simulink model "data_collection_HILS"  (R2024a)
settings: Solver=FixedStepAuto  StartTime=0.0  StopTime=inf  FixedStep=0.01  RelTol=1e-3
libraries: robotlib x6, simulink x2, sharedtransform x1, eeGeneralControl x1
settings Model: Creator=hmcl  LastModifiedBy=yjchun
settings OptimizationCC: EnhancedBackFolding=on  PassReuseOutputArgsAs=Individual arguments  ZeroExternalMemoryAtStartup=off  ZeroInternalMemoryAtStartup=off  MaxStackSize=64  OptimizeBlockOrder=speed  DifferentSizesBufferReuse=on  OptimizationCustomize=off  EfficientTunableParamExpr=on
settings DebuggingCC: ParameterTunabilityLossMsg=error
settings HardwareCC: ProdBitPerPointer=32  ProdBitPerSizeT=32  ProdBitPerPtrDiffT=32  ProdLargestAtomicFloat=None  ProdIntDivRoundTo=Undefined  ProdEndianess=Unspecified  ProdWordSize=32  ProdHWDeviceType=Generic->Unspecified (assume 32-bit Generic)
settings RTWCC: Description=Embedded Coder  SystemTargetFile=ert.tlc  HardwareBoard=Robot Operating System (ROS)  TLCOptions="-aInlineSetEventsForThisBaseRateFcn=TLC_FALSE -aSuppressMultiTaskScheduler=TLC_FALSE  -aRateBasedStepFcn=0"  TemplateMakefile=ert_default_tmf  Toolchain=Catkin  TargetLang=C++  GPUComputeCapability=3.5
settings CodeAppCC: ForceParamTrailComments=on  IgnoreCustomStorageClasses=off  OperatorAnnotations=on  SimulinkDataObjDesc=on  SFDataObjDesc=on  InsertBlockDesc=on

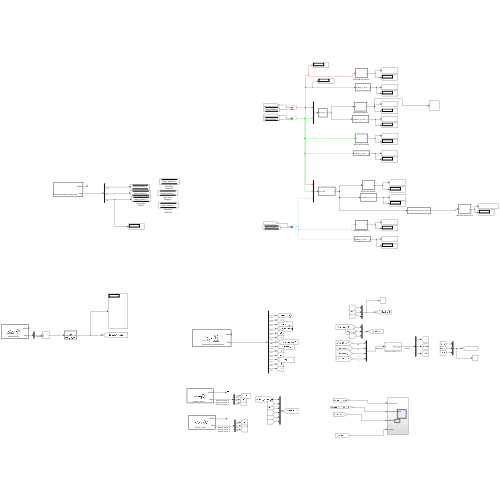
[thumbnail: Simulink's stored preview of the top-level diagram]
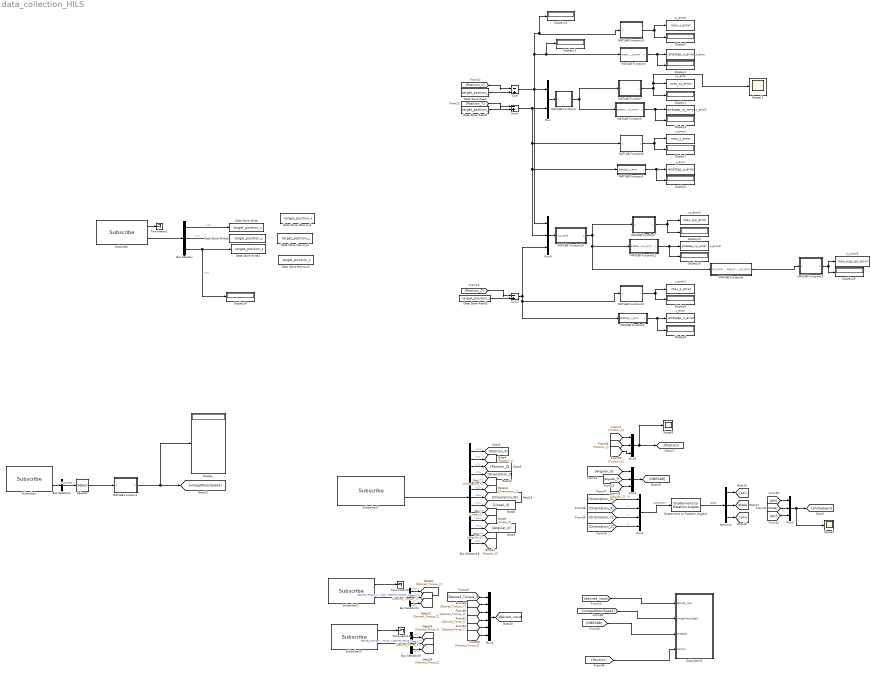
== system data_collection_HILS ==
  Bus Selector : BusSelector  OutputSignals=Pose.Position.X,Pose.Position.Y,Pose.Position.Z
  Bus Selector1 : BusSelector  OutputSignals=Channels
  Bus Selector10 : BusSelector  OutputSignals=X,Y,Z
  Bus Selector11 : BusSelector  OutputSignals=X,Y,Z
  Bus Selector18 : BusSelector  OutputSignals=Pose.Pose.Position.X,Pose.Pose.Position.Y,Pose.Pose.Position.Z,Pose.Pose.Orientation.X,Pose.Pose.Orientation.Y,Pose.Pose.Orientation.Z,Pose.Pose.Orientation.W,Twist.Twist.Linear.X,Twist.Twist.Linear.Y,Twist.Twist.Linear.Z,Twist.Twist.Angular.X,Twist.Twist.Angular.Y,Twist.Twist.Angular.Z
  Data Store Memory3 : DataStoreMemory  DataStoreName=target_position_x  ReadBeforeWriteMsg=warning  WriteAfterWriteMsg=warning  WriteAfterReadMsg=warning  ShowAdditionalParam=off
  Data Store Memory4 : DataStoreMemory  DataStoreName=target_position_y  ReadBeforeWriteMsg=warning  WriteAfterWriteMsg=warning  WriteAfterReadMsg=warning  ShowAdditionalParam=off
  Data Store Memory5 : DataStoreMemory  DataStoreName=target_position_z  ReadBeforeWriteMsg=warning  WriteAfterWriteMsg=warning  WriteAfterReadMsg=warning  ShowAdditionalParam=off
  Data Store Read : DataStoreRead  DataStoreName=target_position_x  IndexOptions=Index vector (dialog)  Indices=1  OutputSizes=1
  Data Store Read1 : DataStoreRead  DataStoreName=target_position_y  IndexOptions=Index vector (dialog)  Indices=1  OutputSizes=1
  Data Store Read3 : DataStoreRead  DataStoreName=target_position_z  IndexOptions=Index vector (dialog)  Indices=1  OutputSizes=1
  Data Store Write : DataStoreWrite  DataStoreName=target_position_x  IndexOptions=Index vector (dialog)  Indices=1  OutputSizes=1
  Data Store Write1 : DataStoreWrite  DataStoreName=target_position_y  IndexOptions=Index vector (dialog)  Indices=1  OutputSizes=1
  Data Store Write2 : DataStoreWrite  DataStoreName=target_position_z  IndexOptions=Index vector (dialog)  Indices=1  OutputSizes=1
  Demux4 : Demux  Outputs=3
  Display{,1..3,5..11,14..16,29} (15 alike) : Display
  MATLAB Function : MATLAB Function  TreatAsAtomicUnit=on
  MATLAB Function1 : MATLAB Function  TreatAsAtomicUnit=on
  MATLAB Function10 : MATLAB Function  TreatAsAtomicUnit=on
  MATLAB Function11 : MATLAB Function  TreatAsAtomicUnit=on
  MATLAB Function12 : MATLAB Function  TreatAsAtomicUnit=on
  MATLAB Function14 : MATLAB Function  TreatAsAtomicUnit=on
  MATLAB Function15 : MATLAB Function  TreatAsAtomicUnit=on
  MATLAB Function2 : MATLAB Function  TreatAsAtomicUnit=on
  MATLAB Function3 : MATLAB Function  TreatAsAtomicUnit=on
  MATLAB Function4 : MATLAB Function  TreatAsAtomicUnit=on
  MATLAB Function5 : MATLAB Function  TreatAsAtomicUnit=on
  MATLAB Function6 : MATLAB Function  TreatAsAtomicUnit=on
  MATLAB Function7 : MATLAB Function  TreatAsAtomicUnit=on
  MATLAB Function8 : MATLAB Function  TreatAsAtomicUnit=on
  MATLAB Function9 : MATLAB Function  TreatAsAtomicUnit=on
  Mux : Mux  Inputs=2
  Mux1 : Mux
  Mux{2..3,5..6} (4 alike) : Mux  Inputs=3
  Mux4 : Mux  Inputs=6
  Quaternions to Rotation Angles1 : sharedtransform/Quaternions to Rotation Angles  rotationOrder=ZYX  aMode=aMode
  Scope11 : Scope
  Scope2 : Scope
  Scope3 : Scope
  Selector : Selector  InputPortWidth=128  IndexOptions=Index vector (dialog)  Indices=1:8  OutputSizes=1
  Subscribe : robotlib/Subscribe  topicSource=Select from ROS network  topic=/mavros/setpoint_position/local  messageType=geometry_msgs/PoseStamped  SampleTime=-1  legacyBusStruct=off  messageQueueLength=1
  Subscribe1 : robotlib/Subscribe  topicSource=Select from ROS network  topic=/mavros/rc/out  messageType=mavros_msgs/RCOut  SampleTime=-1  legacyBusStruct=off  messageQueueLength=1
  Subscribe10 : robotlib/Subscribe  topicSource=Select from ROS network  topic=/thrust_vector  messageType=geometry_msgs/Vector3  SampleTime=-1  legacyBusStruct=off  messageQueueLength=1
  Subscribe11 : robotlib/Subscribe  topicSource=Select from ROS network  topic=/torque_vector  messageType=geometry_msgs/Vector3  SampleTime=-1  legacyBusStruct=off  messageQueueLength=1
  Subscribe17 : robotlib/Subscribe  topicSource=Select from ROS network  topic=/mavros/local_position/odom  messageType=nav_msgs/Odometry  SampleTime=-1  legacyBusStruct=off  messageQueueLength=1
  Subsystem2 : Subsystem
  Sum : Sum  Inputs=|-+
  Sum1 : Sum  Inputs=|-+
  Sum3 : Sum  Inputs=|-+
  Terminator1 : Terminator
  Terminator10 : Terminator
  Terminator11 : Terminator
  x_error : ToWorkspace  VariableName=endstep_x_error  SampleTime=-1
      settings: Save2DSignal=2-D array (concatenate along first dimension)
  x_error1 : ToWorkspace  VariableName=endstep_xy_error  SampleTime=-1
      settings: Save2DSignal=2-D array (concatenate along first dimension)
  x_error2 : ToWorkspace  VariableName=max_y_error  SampleTime=-1
      settings: Save2DSignal=2-D array (concatenate along first dimension)
  x_error3 : ToWorkspace  VariableName=endstep_xyz_error  SampleTime=-1
      settings: Save2DSignal=2-D array (concatenate along first dimension)
  xy_error : ToWorkspace  VariableName=max_xy_error  SampleTime=-1
      settings: Save2DSignal=2-D array (concatenate along first dimension)
  xy_error1 : ToWorkspace  VariableName=max_x_error  SampleTime=-1
      settings: Save2DSignal=2-D array (concatenate along first dimension)
  xy_error2 : ToWorkspace  VariableName=max_xyz_error  SampleTime=-1
      settings: Save2DSignal=2-D array (concatenate along first dimension)
  xy_error3 : ToWorkspace  VariableName=max_avg_xyz_error  SampleTime=-1
      settings: Save2DSignal=2-D array (concatenate along first dimension)
  y_error : ToWorkspace  VariableName=endstep_y_error  SampleTime=-1
      settings: Save2DSignal=2-D array (concatenate along first dimension)
  y_error1 : ToWorkspace  VariableName=max_z_error  SampleTime=-1
      settings: Save2DSignal=2-D array (concatenate along first dimension)
  z_error : ToWorkspace  VariableName=endstep_z_error  SampleTime=-1
      settings: Save2DSignal=2-D array (concatenate along first dimension)
  wires:
  MATLAB Function3/1(y) -> Display6/1, y_error/1
  MATLAB Function2/1(y) -> Display8/1, z_error/1
  MATLAB Function14/1(y) -> xy_error1/1, Display5/1
  MATLAB Function6/1(y) -> x_error2/1, Display7/1
  MATLAB Function/1(y) -> Scope11/1, xy_error/1, Display1/1
  MATLAB Function4/1(y) -> x_error/1, Display2/1
  MATLAB Function11/1(y) -> y_error1/1, Display9/1
  MATLAB Function9/1(y) -> x_error1/1, Display3/1
  Data Store Read/1 -> Sum/2
  Sum3/1 -> MATLAB Function11/1(u), MATLAB Function2/1(endstep_z_error), Mux6/3
  MATLAB Function5/1(y) -> MATLAB Function9/1(endstep_xy_error), MATLAB Function/1(u)
  Data Store Read3/1 -> Sum3/2
  Mux/1 -> MATLAB Function5/1(xy_error)
  Sum/1 -> Mux6/1, MATLAB Function14/1(u), Display10/1, Display11/1, MATLAB Function4/1(endstep_x_error), Mux/1
  Sum1/1 -> Mux6/2, MATLAB Function3/1(endstep_y_error), MATLAB Function6/1(u), Mux/2
  Data Store Read1/1 -> Sum1/2
  [Orientation_W] -> Mux1/1  "W"
  Demux4/3 -> [phi]
  Demux4/1 -> [psi]
  Demux4/2 -> [theta]
  [Orientation_Y] -> Mux1/3  "Y"
  Quaternions to Rotation Angles1/1 -> Demux4/1  "radian"
  [Orientation_X] -> Mux1/2  "x"
  [Orientation_Z] -> Mux1/4  "z"
  Mux1/1 -> Quaternions to Rotation Angles1/1  "quertanion"
  [phi] -> Mux2/1
  Mux2/1 -> Scope2/1, [phithetapsi]
  [psi] -> Mux2/3
  [theta] -> Mux2/2
  [Position_X] -> Sum/1
  [Position_Y] -> Sum1/1
  [Position_Z] -> Sum3/1
  [Angular_X] -> Mux3/1
  [Angular_Y] -> Mux3/2
  [Angular_Z] -> Mux3/3
  Mux3/1 -> [OMEGAB]
  [OMEGAB] -> Subsystem2/3(OMEGAB)
  [desired_input] -> Subsystem2/1(desired_input)
  [omegaMotorSpeed] -> Subsystem2/2(omegaMotorSpeed)
  [Desired_Force_X] -> Mux4/4
  [Desired_Torque_Y] -> Mux4/2
  Bus Selector11/3 -> [Desired_Torque_Z]  "<Z>"
  [Desired_Torque_X] -> Mux4/1
  Subscribe10/1 -> Terminator11/1
  Subscribe11/2 -> Bus Selector11/1  "Desired_Torque_X Desired_Torque_Y Desired_Torque_Z"
  [Desired_Torque_Z] -> Mux4/3
  [Desired_Force_Y] -> Mux4/5
  [Desired_Force_Z] -> Mux4/6
  Subscribe11/1 -> Terminator10/1
  Bus Selector10/3 -> [Desired_Force_Z]  "<Z>"
  Bus Selector10/2 -> [Desired_Force_Y]  "<Y>"
  Subscribe10/2 -> Bus Selector10/1  "Desired_Force_X Desired_Force_Y Desired_Force_Z"
  Bus Selector11/1 -> [Desired_Torque_X]  "<X>"
  Bus Selector11/2 -> [Desired_Torque_Y]  "<Y>"
  Bus Selector10/1 -> [Desired_Force_X]  "<X>"
  Mux4/1 -> [desired_input]
  [Position_X] -> Mux5/1
  [Position_Y] -> Mux5/2
  [Position_Z] -> Mux5/3
  Mux5/1 -> Scope3/1, [Position]
  Mux6/1 -> MATLAB Function10/1(xyz_error)
  MATLAB Function10/1(y) -> MATLAB Function7/1(u), MATLAB Function8/1(xyz_error), MATLAB Function12/1(endstep_xyz_error)
  MATLAB Function7/1(y) -> xy_error2/1, Display15/1
  MATLAB Function12/1(y) -> x_error3/1, Display16/1
  Subscribe17/2 -> Bus Selector18/1
  Bus Selector18/1 -> [Position_X]  "<X>"
  Bus Selector18/2 -> [Position_Y]  "<Y>"
  Bus Selector18/3 -> [Position_Z]  "<Z>"
  Bus Selector18/4 -> [Orientation_X]  "<X>"
  Bus Selector18/5 -> [Orientation_Y]  "<Y>"
  Bus Selector18/6 -> [Orientation_Z]  "<Z>"
  Bus Selector18/7 -> [Orientation_W]  "<W>"
  Bus Selector18/8 -> [Linear_X]  "<X>"
  Bus Selector18/9 -> [Linear_Y]  "<Y>"
  Bus Selector18/10 -> [Linear_Z]  "<Z>"
  Bus Selector18/11 -> [Angular_X]  "<X>"
  Bus Selector18/12 -> [Angular_Y]  "<Y>"
  Bus Selector18/13 -> [Angular_Z]  "<Z>"
  [Position] -> Subsystem2/4(Position)
  MATLAB Function8/1(avg_array_xyz_error) -> MATLAB Function15/1(u)
  MATLAB Function15/1(y) -> xy_error3/1, Display29/1
  Bus Selector/3 -> Display14/1, Data Store Write2/1  "<Z>"
  Bus Selector/1 -> Data Store Write/1  "<X>"
  Subscribe/1 -> Terminator1/1
  Bus Selector/2 -> Data Store Write1/1  "<Y>"
  Subscribe/2 -> Bus Selector/1
  MATLAB Function1/1(rad_s_out) -> Display/1, [omegaMotorSpeed]
  Subscribe1/2 -> Bus Selector1/1
  Selector/1 -> MATLAB Function1/1(pwm_in)
  Bus Selector1/1 -> Selector/1  "<Channels>"

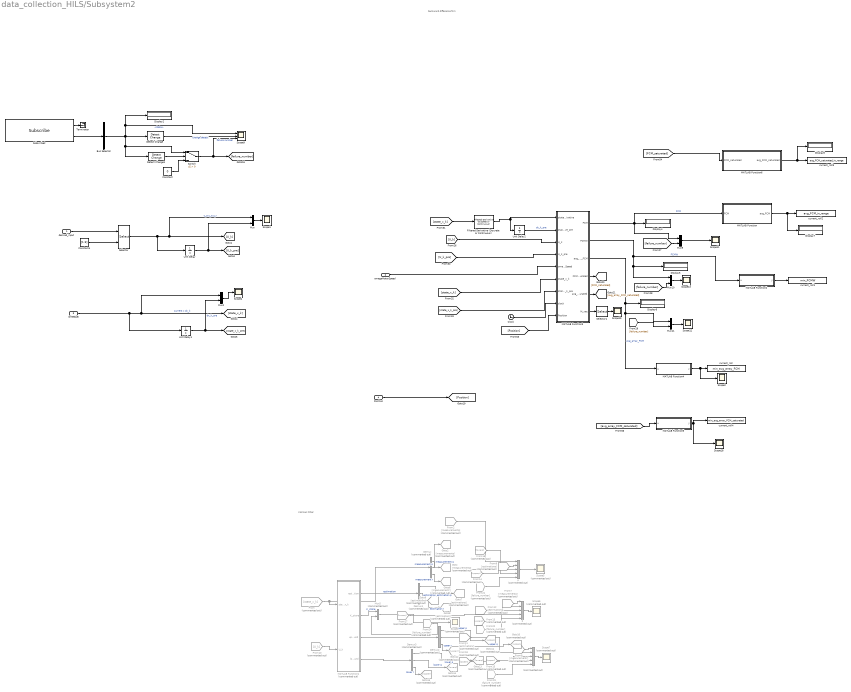
== system data_collection_HILS/Subsystem2 ==
  note: Kalman Filter
  note: backward difference fcm
  desired_input : Inport
  omegaMotorSpeed : Inport  Port=2
  OMEGAB : Inport  Port=3
  Position : Inport  Port=4
  Bus Selector : BusSelector  OutputSignals=Data
  Clock : Clock
  Constant : Constant  Value=0
  Constant4 : Constant  Value=[1:3]
  Demux{,1..3} (4 alike) : Demux  Commented=on  Outputs=3
  Detect Change : simulink/Logic and Bit Operations/Detect Change  vinit=0  OutDataTypeStr=boolean
  Detect Change1 : simulink/Logic and Bit Operations/Detect Change  vinit=0  OutDataTypeStr=boolean
  Display{2,4..8} (6 alike) : Display
  Filtered Derivative (Discrete or Continuous) : eeGeneralControl/Filtered Derivative (Discrete or Continuous)  K=1  T=0.1  B=inf  A=-inf  minRatio=10  init_option=Inherited from block input  x0=0  Ts=-1
      settings: LibrarySourceBlock=|
      | ee_sl_lib/General Control/Filtered Derivative
      | (Discrete or Continuous)
  From : From  Commented=on  GotoTag=state_x_k
  From10 : From  Commented=on  GotoTag=U_k
  From11 : From  Commented=on  GotoTag=estimationr
  From12 : From  Commented=on  GotoTag=estimationq
  From13 : From  Commented=on  GotoTag=upperq
  From14 : From  Commented=on  GotoTag=upperp
  From15 : From  Commented=on  GotoTag=upperr
  From16 : From  Commented=on  GotoTag=lowerp
  From17 : From  Commented=on  GotoTag=lowerq
  From18 : From  Commented=on  GotoTag=lowerr
  From2 : From  Commented=on  GotoTag=measurementp
  From{21..24} (4 alike) : From  Commented=on  GotoTag=failure_number
  From7 : From  Commented=on  GotoTag=measurementq
  From8 : From  Commented=on  GotoTag=measurementr
  From9 : From  Commented=on  GotoTag=estimationp
  Goto : Goto  Commented=on  GotoTag=measurementp
  Goto10 : Goto  Commented=on  GotoTag=upperq
  Goto11 : Goto  Commented=on  GotoTag=upperp
  Goto12 : Goto  Commented=on  GotoTag=upperr
  Goto13 : Goto  Commented=on  GotoTag=lowerp
  Goto14 : Goto  Commented=on  GotoTag=lowerq
  Goto15 : Goto  Commented=on  GotoTag=lowerr
  Goto2 : Goto  Commented=on  GotoTag=measurementq
  Goto6 : Goto  Commented=on  GotoTag=measurementr
  Goto7 : Goto  Commented=on  GotoTag=estimationp
  Goto8 : Goto  Commented=on  GotoTag=estimationr
  Goto9 : Goto  Commented=on  GotoTag=estimationq
  MATLAB Function : MATLAB Function  TreatAsAtomicUnit=on
  MATLAB Function1 : MATLAB Function  Commented=on  TreatAsAtomicUnit=on
  MATLAB Function2 : MATLAB Function  TreatAsAtomicUnit=on
  MATLAB Function3 : MATLAB Function  TreatAsAtomicUnit=on
  MATLAB Function4 : MATLAB Function  TreatAsAtomicUnit=on
  MATLAB Function5 : MATLAB Function  TreatAsAtomicUnit=on
  MATLAB Function6 : MATLAB Function  TreatAsAtomicUnit=on
  Mux{,2,9..11} (5 alike) : Mux  Inputs=2
  Mux5 : Mux  Commented=on  Inputs=2
  Scope{1..2,4,11..13,18..19} (8 alike) : Scope
  Scope{5..8} (4 alike) : Scope  Commented=on
  Scope9 : Scope  NumInputPorts=3
  Selector : Selector  InputPortWidth=6  IndexOptions=Index vector (port)  Indices=[1 3]  OutputSizes=1
  Selector1 : Selector  InputPortWidth=9  IndexOptions=Index vector (dialog)  Indices=[1 5 9]  OutputSizes=1
  Subscribe2 : robotlib/Subscribe  topicSource=Select from ROS network  topic=/mavros/keyboard_command/failure_number  messageType=std_msgs/Float32  SampleTime=-1  legacyBusStruct=off  messageQueueLength=1
  Switch : Switch  Criteria=u2 > Threshold  SaturateOnIntegerOverflow=off  InputSameDT=off
  Terminator : Terminator
  Unit Delay : UnitDelay  SampleTime=-1  HasFrameUpgradeWarning=on
  Unit Delay1 : UnitDelay  SampleTime=-1  HasFrameUpgradeWarning=on
  Unit Delay2 : UnitDelay  SampleTime=-1  HasFrameUpgradeWarning=on
  current_roll : ToWorkspace  VariableName=min_avg_array_FCM  SampleTime=-1
      settings: Save2DSignal=2-D array (concatenate along first dimension)
  current_roll1 : ToWorkspace  VariableName=min_FCMW  SampleTime=-1
      settings: Save2DSignal=2-D array (concatenate along first dimension)
  current_roll2 : ToWorkspace  VariableName=avg_FCM_in_range  SampleTime=-1
      settings: Save2DSignal=2-D array (concatenate along first dimension)
  current_roll3 : ToWorkspace  VariableName=avg_FCM_saturated_in_range  SampleTime=-1
      settings: Save2DSignal=2-D array (concatenate along first dimension)
  current_roll4 : ToWorkspace  VariableName=min_avg_array_FCM_saturated  SampleTime=-1
      settings: Save2DSignal=2-D array (concatenate along first dimension)
  p : Mux  Commented=on  Inputs=5
  q : Mux  Commented=on  Inputs=5
  r : Mux  Commented=on  Inputs=5
  wires:
  desired_input/1 -> Selector/1
  Unit Delay/1 -> Mux/2, [U_k_pre]
  OMEGAB/1 -> Mux2/1, [state_x_k], Unit Delay1/1  "current x dx_k"
  Unit Delay1/1 -> Mux2/2, [state_x_k_pre]  "dx_k_pre"
  Constant4/1 -> Selector/2
  Selector/1 -> Mux/1, [U_k], Unit Delay/1  "u_p u_q u_r"
  Mux/1 -> Scope1/1
  Mux2/1 -> Scope4/1
  Subscribe2/1 -> Terminator/1
  Subscribe2/2 -> Bus Selector/1
  Bus Selector/1 -> Switch/1, Detect Change1/1, Scope9/1, Display2/1, Detect Change/1  "<Data>"
  Detect Change/1 -> Scope9/2  "change detect"
  Detect Change1/1 -> Switch/2
  Switch/1 -> [failure_number], Scope9/3  "failure number"
  Constant/1 -> Switch/3
  [failure_number] -> Mux9/2
  Mux11/1 -> Scope12/1
  MATLAB Function3/2(FCMW) -> Mux10/1, Display5/1, MATLAB Function2/1(u)  "FCMW"
  [state_x_k] -> Filtered Derivative (Discrete or Continuous)/1
  [U_k_pre] -> MATLAB Function3/4(U_k_pre)
  Mux10/1 -> Scope13/1
  [state_x_k] -> MATLAB Function3/6(state_x_k)
  [failure_number] -> Mux10/2
  Mux9/1 -> Scope11/1
  MATLAB Function3/3(avg_array_FCM) -> MATLAB Function4/1(u), Mux11/1, Display6/1  "avg_array_FCM"
  [failure_number] -> Mux11/2
  MATLAB Function3/1(FCM) -> MATLAB Function/1(FCM), Display4/1, Mux9/1  "FCM"
  [U_k] -> MATLAB Function3/3(U_k)
  omegaMotorSpeed/1 -> MATLAB Function3/5(omegaMotorSpeed)
  [state_x_k_pre] -> MATLAB Function3/7(state_x_k_pre)
  Demux1/3 -> Goto8/1  "estimation r"
  MATLAB Function1/1(estimation) -> Demux1/1  "estimation"
  MATLAB Function1/4(lower_bound) -> Demux3/1
  From2/1 -> p/1
  From13/1 -> q/3
  From21/1 -> p/5
  From12/1 -> q/2
  From16/1 -> p/4
  Demux/1 -> Goto/1  "measurement p"
  Demux1/2 -> Goto9/1  "estimation q"
  Demux3/2 -> Goto14/1  "lower q"
  q/1 -> Scope6/1
  From18/1 -> r/4
  Demux1/1 -> Goto7/1  "estimation p"
  r/1 -> Scope7/1
  From23/1 -> r/5
  Demux/2 -> Goto2/1  "measurement q"
  Demux2/2 -> Goto10/1  "upper q"
  From9/1 -> p/2
  From/1 -> Demux/1, MATLAB Function1/1(state_x_k)
  From14/1 -> p/3
  Demux3/3 -> Goto15/1  "lower r"
  Demux3/1 -> Goto13/1  "lower p"
  Demux2/1 -> Goto11/1  "upper p"
  From22/1 -> q/5
  From10/1 -> MATLAB Function1/2(U_k)
  From11/1 -> r/2
  From24/1 -> Mux5/2
  From7/1 -> q/1
  p/1 -> Scope5/1
  From17/1 -> q/4
  MATLAB Function1/3(upper_bound) -> Demux2/1
  Demux/3 -> Goto6/1  "measurement r"
  MATLAB Function1/2(K_store) -> Mux5/1  "K_store"
  From15/1 -> r/3
  Mux5/1 -> Scope8/1
  From8/1 -> r/1
  Demux2/3 -> Goto12/1  "upper r"
  MATLAB Function4/1(y) -> current_roll/1, Scope2/1
  MATLAB Function2/1(y) -> current_roll1/1
  Filtered Derivative (Discrete or Continuous)/1 -> Unit Delay2/1, MATLAB Function3/1(state_derivative)
  MATLAB Function/1(avg_FCM) -> current_roll2/1, Display7/1
  Clock/1 -> MATLAB Function3/8(clock)
  Position/1 -> [Position]
  [FCM_saturated] -> MATLAB Function6/1(FCM_saturated)
  MATLAB Function6/1(avg_FCM_saturated) -> Display8/1, current_roll3/1
  [Position] -> MATLAB Function3/9(Position)
  MATLAB Function3/4(FCM_saturated) -> [FCM_saturated]
  MATLAB Function3/5(avg_array_FCM_saturated) -> [avg_array_FCM_saturated]
  MATLAB Function5/1(y) -> current_roll4/1, Scope18/1
  [avg_array_FCM_saturated] -> MATLAB Function5/1(u)
  MATLAB Function3/6(M_vec) -> Selector1/1
  Selector1/1 -> Scope19/1
  Unit Delay2/1 -> MATLAB Function3/2(state_derivative_pre)  "dx_k_pre"

== matlab function data_collection_HILS/Subsystem2/MATLAB Function ==
  data: FCM input; avg_FCM output
function avg_FCM = fcn(FCM)
% HILS 환경에서는 전체 시뮬레이션 시간 동안의 누적 평균을 계산합니다.

    coder.extrinsic('assignin'); 
    persistent total_sum total_count;

    % persistent 변수 초기화
    if isempty(total_sum)
        total_sum = 0;
    end
    if isempty(total_count)
        total_count = 0;
    end

    % 매 스텝마다 합계와 카운트를 누적
    total_sum = total_sum + FCM;
    total_count = total_count + 1;

    % 현재까지의 평균 계산 (0으로 나누는 오류 방지)
    if total_count > 0
        avg_FCM = total_sum / total_count;
    else
        avg_FCM = 0; % 초기값은 0으로 설정
    end
    
    % 계산된 평균값을 MATLAB Workspace의 'avg_FCM_in_range' 변수에 실시간으로 전송
    assignin('base', 'avg_FCM_in_range', avg_FCM);

end

== matlab function data_collection_HILS/Subsystem2/MATLAB Function1 ==
  data: state_x_k input; estimation output; U_k input; K_store output; upper_bound output; lower_bound output
function [estimation, K_store,upper_bound, lower_bound]  = fcn(state_x_k, U_k)

%% Extended Kalman Filter Example
%% Initial Conditions
coder.extrinsic('delft_evaluate_jacobians');
coder.extrinsic('size');
coder.extrinsic('norm');
coder.extrinsic('eye');
coder.extrinsic('diag');
coder.extrinsic('subs');
coder.extrinsic('calculate_dynamics');
% persistent 변수 선언
persistent initialized xp Pp;

% 초기화가 필요할 때만 실행
if isempty(initialized)
    initialized = true; % 초기화 완료 표시
    xp = state_x_k;    % guess of initial posteriori estimation
    Pp = 100*eye(3); % guess of initial error covariance
    sigma_Pp = sqrt(diag(Pp));
    three_sigma = zeros(3,1);
    upper_bound = zeros(3,1);
    lower_bound = zeros(3,1);

    P = zeros(3,3);


    x_ = zeros(3,1);
    P_ = zeros(3,3);
    Pp_ = zeros(3,3);
    F = zeros(3,3);
    Q = zeros(3,3);
    R = zeros(3,3);
    K = zeros(3,3);
    H = zeros(3,3);
    I = zeros(3,3);
    estimation = zeros(3,1);
    K_store = zeros(1,1);
    disp('initialized.');
end

p = xp(1);
q = xp(2);
r = xp(3);

u_p = U_k(1);
u_q = U_k(2);
u_r = U_k(3);

sigma_w = 0.1;      % system noise (std of acceleration)
sigma_v = 0.2;      % measurement noise (std of position sensor)
Q = diag([sigma_w^2 sigma_w^2 sigma_w^2]); % system noise covariance matrix
R = diag([sigma_v^2 sigma_v^2 sigma_v^2]); % measurement noise covariance matrix
%% Dynamics
% system matrix

Gamma = [1 0 0;0 1 0;0 0 1];      % Gamma (related to system noise)
H = [1 0 0;0 1 0;0 0 1];          % Measurement matrix

%% KF Routine
    %% True dynamics
    % x(:,i+1) = [sin(x(2,i)*(i)) + randn*sigma_w; x(2,i) ]; % system dynamics
    % x = double(subs(F, {'p', 'q', 'r','u_p', 'u_q', 'u_r'},{p, q, r, u_p, u_q, u_r}));
    %% ====================================================
    %% Time update
    %% ====================================================
    %% Equation 1: Prediction of state
    % x_ = [sin(xp(2,i)*(i)); xp(2,i)];
    x_ = calculate_dynamics(p, q, r, u_p, u_q, u_r);
    %% compute Jacobian
    % F = [0 (i)*cos(x_(2)*(i));
    %     0 1];
    [F_, G_] = delft_evaluate_jacobians(p, q, r, u_p, u_q, u_r);
    %% Equation 2: Prediction of covariance
    F = F_;
    Pp_ = Pp;
    P_ = F*Pp_*F' + Gamma*Q*Gamma';
    %% ====================================================
    %% Measurement update
    %% ====================================================
    %% measurement generation
    % y(i) = H*x(:,i+1) + randn*sigma_v;
    y = state_x_k;
    %% Equation 3: Innovation Covariance
    S = H*P_*H'+R;
    %% Equation 4:  Residual
    nu = y-H*x_;
    %% Equation 5: Kalman gain
    K = P_*H'*S^-1;
    %% Equation 6: State update
    xp = x_ + K * nu;
    estimation = xp;
    %% Equation 7: Covariance update
    I = eye(size(K*H));
    Pp = (I-K*H)*P_;
    %% =====================================================
    %% storing error covariance for ploting
    sigma_Pp = sqrt(diag(Pp));
    % disp('sigma_Pp');
    % disp(size(sigma_Pp));
    three_sigma = 3 * sigma_Pp;
    upper_bound = xp + three_sigma;
    lower_bound = xp - three_sigma;
    %% storing Kalman gain for ploting
    K_store = norm(K);


    
%     %% Plot: position estimate x_1
% figure(1); clf; hold on;
% plot(t,x(1,:),'-b');                  % plot the real plant behavior
% plot(t(1:end-1),y,'.m');                       % plot the observations over this plant
% plot(t,xp(1,:),'-r');                 % plot the Kalman filter prediction over the plant
% plot(t,xp(1,:)+3*sigma_Pp(1,:),':k');  % The threshold in which the true state is
% plot(t,xp(1,:)-3*sigma_Pp(1,:),':k');
% xlabel('time, s'); ylabel('x1: m')
% legend('real','observation','KF','threshold')
% axis([-inf inf -10 10])
% %% Plot: velocity estimate x_2
% figure(2); clf; hold on;
% plot(t,x(2,:),'-b');                  % plot the real plant behavior
% plot(t,xp(2,:),'-r');                 % plot the Kalman filter prediction over the plant
% plot(t,xp(2,:)+3*sigma_Pp(2,:),':k');   % These two are the threshold in witch I'm certain that the plant state is at a given time
% plot(t,xp(2,:)-3*sigma_Pp(2,:),':k');
% xlabel('time, s'); ylabel('x2: rad/s')
% legend('true','KF','threshold')
% axis([-inf inf -5 20])
% %% Plot: Kalman gain norm
% figure(3);
% plot(t(1:end-1),K_store);
% xlabel('time, s'); ylabel('Kalman gain norm')

end

== matlab function data_collection_HILS/Subsystem2/MATLAB Function2 ==
  data: u input; y output
function y = fcn(u)
    coder.extrinsic('assignin');
    persistent min_val; % 최솟값을 저장할 변수

    if isempty(min_val)
        min_val = inf; % 처음에 매우 큰 값으로 초기화
    end

    % 현재 u의 절대값이 기록된 최솟값보다 작으면 업데이트
    if abs(u) < min_val
        min_val = abs(u);
    end

    y = min_val; % 현재까지의 최솟값을 출력
    assignin('base', 'min_avg_array_FCM_saturated', y);
end

== matlab function data_collection_HILS/Subsystem2/MATLAB Function3 ==
  settings: updateMethod=DISCRETE
  data: state_derivative input; state_derivative_pre input; U_k input; U_k_pre input; FCM output; omegaMotorSpeed input; state_x_k input; state_x_k_pre input; FCMW output; avg_array_FCM output; clock input; Position input; FCM_saturated output; avg_array_FCM_saturated output; window_size_ parameter; M_vec output size=9
function [FCM, FCMW, avg_array_FCM, FCM_saturated, avg_array_FCM_saturated,M_vec]  = fcn(state_derivative,state_derivative_pre,U_k,U_k_pre,omegaMotorSpeed,state_x_k,state_x_k_pre,clock, Position, window_size_)
%#codegen

% X_k = current
% X_k_pre = previous
disp('clock = ');
disp(clock);

coder.extrinsic('size');
coder.extrinsic('ctrb');
coder.extrinsic('rank');
coder.extrinsic('inv');
coder.extrinsic('sign');
coder.extrinsic('evalin');
coder.extrinsic('diff');
coder.extrinsic('addpath');
% addpath('/home/hmcl/PX4_testbed/gp_matlab/octo_model');

coder.extrinsic('delft_evaluate_jacobians.m');
coder.extrinsic('calculate_FCMW.m');
coder.extrinsic('calculate_FCMW_saturated.m')

% persistent 변수 선언
persistent initialized avg_array_FCM_ avg_array_FCM_saturated_;
persistent M_prev;

if isempty(M_prev)
    M_prev = eye(3);
end


dt = 0.004; % 시간 간격 % 가제보는 dt = 0.004 로 데이터를 전송및 한다
omega_max = 425.47; % 최대 회전 속도 rad/s, maxRotVelocity in sdf
tau = 0.01; % 액추에이터 시간 상수
M = eye(3);
% window_size_ = 100;

delft_df_dx = zeros(length(state_x_k), length(state_x_k));
delft_df_du = zeros(length(state_x_k), length(U_k));
del_umax = zeros(3,1);
del_uc = zeros(3,1);
signMask = zeros(1,8);
refOmega = zeros(8,1);
signError = zeros(1,1);
rank_con = 0;


rotorMapping = [-1 -1 1;
    1 1 1;
    -1 -1 -1;
    -1 1 -1;
    1 -1 -1;
    1 1 -1;
    1 -1 1;
    -1 1 1];

% rotorMapping = rotorMapping *-1; 

% x = state_x_k1(1);
% y = state_x_k1(2);
% z = state_x_k1(3);
% u = state_x_k1(4);
% v = state_x_k1(5);
% w = state_x_k1(6);
% phi = state_x_k1(7);
% theta = state_x_k1(8);
% psi = state_x_k1(9);
p = state_x_k(1);
q = state_x_k(2);
r = state_x_k(3);

u_p = U_k(1);
u_q = U_k(2);
u_r = U_k(3);

x = Position(1);
y = Position(2);
z = Position(3);



% 초기화가 필요할 때만 실행
if isempty(initialized)
    initialized = true; % 초기화 완료 표시
    FCMW = 1;
    avg_array_FCM = 1.0;
    avg_array_FCM_ = 1.0;

    FCMW_saturated = 1;
    avg_array_FCM_saturated = 1.0;
    avg_array_FCM_saturated_ = 1.0;
    disp('initialized.');
end

disp('-----------------');
% 심볼릭 야코비안 행렬 평가
[df_dx_temp, df_du_temp] = delft_evaluate_jacobians(p, q, r, u_p, u_q, u_r);

% 외부 함수로부터 받은 값을 MATLAB 배열로 변환
delft_df_dx = df_dx_temp; %delft_df_dx = A %3by3   %length(X_k1) by length(X_k1)

delft_df_du = df_du_temp; %delft_df_du = B %3by3    %length(X_k1) by length(U_k1)

A = delft_df_dx;
B = delft_df_du;

debug_info = struct(); 
debug_info.clock = clock;
debug_info.A = A;
debug_info.B_initial = B; 

% 상태 및 입력 차이 계산
diffrate = state_x_k - state_x_k_pre;  % dx는 3x1
du = U_k - U_k_pre;  % du는 3x1

diff_ratedot = state_derivative - state_derivative_pre;




% disp('A = ')
% disp(A)
% disp('du = ')
% disp(du)

% dx_dot = df_dx * dx + df_du * du;
%{
state X 가 정확값이라고 했을때 state X를 미분하면 dx_dot 이 나오게 된다.
그리고 식(6)을 보면 dx_dot 을 근사한 식인 A * dx + B * du 가 있다.
만약 근사한식이 너무 정확하면 dx_dot - (A * dx + B * du) 을 했을때 0 이 된다.
즉, 근사한 식이 정확하면 미분한 식(dx_dot) - 근사한식(A * dx + B * du) 이 0이 되야한다.

하지만 근사한식이 당연히 정확할수 없기 때문에 error가 생기는데
이 에러를 보상해주기 위해, 또는 0으로 수렴 시키기 위해서
del_uc를 정의 해준다.
del_uc는 inv(B) *error 이다.

그래서 dx_dot - (A * dx + B * du + del_uc) 식(11)이 나오고 이 식은 0으로 점점 수렴하게 된다.
%}

error = diff_ratedot - A * diffrate;
debug_info.ER = error; % M 계산에 사용되는 error

M = M_prev; 

% corrcoef_result = corrcoef(state_derivative, A * dx + B * du);
corrcoef_result = corrcoef(diff_ratedot, B * du);

disp('error = ')
disp(error);
disp('B * du = ')
disp(B * du);

for i = 1:3
    if ~isnan(corrcoef_result(1,2))
        M(i, i) = max(corrcoef_result(1,2), 0.001); % 최소값 설정
    else
        M(i, i) = 1;
    end
end
debug_info.corrcoef_result = corrcoef_result;                                                 
debug_info.M = M;

% disp('ER = ')
% disp(error)
% disp('M = ');
% disp(M);
M_vec = M(:);

disp('corrcoef_result = ')
disp(corrcoef_result);

% disp('B = ')
% disp(B)

B = B * M;
debug_info.B_updated = B; % M을 곱한 후 B


M_prev = M;

% disp('B = ')
% disp(B)


% disp('A * dx + B * du = ');
% disp(A * diffrate + B * du);

err = error - B * du; %error : 3by1
% disp('error = ');
% disp(err);
debug_info.err_final = err; % del_uc 계산에 사용되는 최종 error

if (abs(err) == 0)
    
    disp('error is zero');
    FCM = 1;
    FCMW = 1;
    FCM_saturated = 1;

    FCMW_saturated = 1;
    avg_array_FCM = avg_array_FCM_;
    avg_array_FCM_saturated = avg_array_FCM_saturated_;
    return

else
    del_uc = (inv(B)) * err; % del_uc는 3x1
debug_info.del_uc_abs = abs(del_uc);


    rotorMapping_T = rotorMapping'; % 이건 필수인듯?



    % error의 부호를 계산
    for i = 1:length(err)

        signError = sign(err(i));

        signMask = signError .* rotorMapping_T(i,:); % sign(error)를 대체
 

        for j = 1:length(signMask)
            if signMask(j) < 0
                refOmega(j) = omega_max; % signMask가 0보다 작으면 omega_max 할당
            else
                refOmega(j) = 0;         % signMask가 0 이상이면 0 할당
            end
        end

   

        % omegaMotorSpeed [rad/s]
        maxDiff = abs(abs(double(omegaMotorSpeed)) - refOmega); %maxDiff  8by1
  

        % Δu_MAX
        del_umax(i,1) = dt * (1/tau) * sum(maxDiff);

    end
        debug_info.del_umax = del_umax;



    controllability_matrix = ctrb(A,B);
    % disp('controllability_matrix = ')
    % disp(controllability_matrix)

    % 랭크 계산
    rank_con = rank(controllability_matrix);
debug_info.rank = rank_con;

    n = length(A);

 

    if rank_con < n || any(del_umax < abs(del_uc))
        FCM = 0;
    else
        FCM = 1;
    end

if FCM == 0
    fprintf('\n--- FCM=0 DETECTED (Clock: %f) ---\n', debug_info.clock);
    disp('Initial A Matrix:');
    disp(debug_info.A);
    disp('Initial B Matrix:');
    disp(debug_info.B_initial);
    disp('ER (for M calculation):');
    disp(debug_info.ER)

      disp('corrcoef_result:');
    disp(debug_info.corrcoef_result)
    
    disp('Calculated M Matrix:');
    disp(debug_info.M);
    disp('Updated B Matrix (B*M):');
    disp(debug_info.B_updated);
    disp('Final Error (for del_uc):');
    disp(debug_info.err_final);
    disp('Required Control |del_uc|:');
    disp(debug_info.del_uc_abs);
    disp('Max Available Control |del_umax|:');
    disp(debug_info.del_umax);
    disp('Controllability Matrix Rank:');
    disp(debug_info.rank);
    fprintf('-------------------------------------\n\n');
end



    [FCMW_, avg_array_FCM_] = calculate_FCMW(FCM,window_size_);

    FCMW = FCMW_;
    avg_array_FCM = avg_array_FCM_;



    if sqrt(x^2 + y^2) < 10
        FCM_saturated = FCM;
    else
        FCM_saturated = 0;
    end

    [FCMW_saturated_, avg_array_FCM_saturated_] = calculate_FCMW_saturated(FCM_saturated,window_size_);

    FCMW_saturated = FCMW_saturated_;
    avg_array_FCM_saturated = avg_array_FCM_saturated_;


end % if end

disp('-----------------');

end

== matlab function data_collection_HILS/MATLAB Function10 ==
  data: xyz_error input; y output
function y = two_norm(xyz_error)
    coder.extrinsic('norm'); % MATLAB 함수 사용을 알림
    
    

    
    % 'y'를 명확히 초기화
    y = 0; 
    
y = norm(xyz_error,2);

== matlab function data_collection_HILS/MATLAB Function11 ==
  data: u input; y output
function y = fcn(u)
% HILS 환경에서는 전체 시뮬레이션 시간 동안 u의 최댓값을 찾습니다.

    coder.extrinsic('assignin');
    persistent max_val; % 최댓값을 저장할 변수

    % persistent 변수 초기화
    if isempty(max_val)
        max_val = -inf; % 처음에 매우 작은 값으로 초기화
    end

    % 현재 u가 기록된 최댓값보다 크면 업데이트
    if u > max_val
        max_val = u;
    end

    y = max_val; % 현재까지의 최댓값을 출력
    
    % 계산된 최댓값을 MATLAB Workspace 변수에 실시간으로 전송
    assignin('base', 'max_z_error', y);

end

== matlab function data_collection_HILS/MATLAB Function12 ==
  data: endstep_xyz_error input; y output
function y = fcn(endstep_xyz_error)

% z_error 값을 기본 워크스페이스에 저장
assignin('base', 'endstep_xyz_error', endstep_xyz_error);

% 저장된 값을 반환
y = endstep_xyz_error;

end

== matlab function data_collection_HILS/MATLAB Function14 ==
  data: u input; y output
function y = fcn(u)
% HILS 환경에서는 전체 시뮬레이션 시간 동안 u의 최댓값을 찾습니다.

    coder.extrinsic('assignin');
    persistent max_val; % 최댓값을 저장할 변수

    % persistent 변수 초기화
    if isempty(max_val)
        max_val = -inf; % 처음에 매우 작은 값으로 초기화
    end

    % 현재 u가 기록된 최댓값보다 크면 업데이트
    if u > max_val
        max_val = u;
    end

    y = max_val; % 현재까지의 최댓값을 출력
    
    % 계산된 최댓값을 MATLAB Workspace 변수에 실시간으로 전송
    assignin('base', 'max_x_error', y);

end

== matlab function data_collection_HILS/Subsystem2/MATLAB Function5 ==
  data: u input; y output
function y = fcn(u)
% HILS 환경에서는 전체 시뮬레이션 시간 동안 u의 절대값 최솟값을 찾습니다.

    coder.extrinsic('assignin');
    persistent min_val; % 최솟값을 저장할 변수

    % persistent 변수 초기화
    if isempty(min_val)
        min_val = inf; % 처음에 매우 큰 값으로 초기화
    end

    % 현재 u의 절대값이 기록된 최솟값보다 작으면 업데이트
    if abs(u) < min_val
        min_val = abs(u);
    end

    y = min_val; % 현재까지의 최솟값을 출력
    
    % 계산된 최솟값을 MATLAB Workspace 변수에 실시간으로 전송
    assignin('base', 'min_avg_array_FCM_saturated', y);

end

== matlab function data_collection_HILS/Subsystem2/MATLAB Function6 ==
  data: FCM_saturated input; avg_FCM_saturated output
function avg_FCM_saturated = fcn(FCM_saturated)
% HILS 환경에서는 전체 시뮬레이션 시간 동안의 누적 평균을 계산합니다.

    coder.extrinsic('assignin'); 
    persistent total_sum total_count;

    % persistent 변수 초기화
    if isempty(total_sum)
        total_sum = 0;
    end
    if isempty(total_count)
        total_count = 0;
    end

    % 매 스텝마다 합계와 카운트를 누적
    total_sum = total_sum + FCM_saturated;
    total_count = total_count + 1;

    % 현재까지의 평균 계산 (0으로 나누는 오류 방지)
    if total_count > 0
        avg_FCM_saturated = total_sum / total_count;
    else
        avg_FCM_saturated = 0; % 초기값은 0으로 설정
    end
    
    % 계산된 평균값을 MATLAB Workspace 변수에 실시간으로 전송
    assignin('base', 'avg_FCM_saturated_in_range', avg_FCM_saturated);

end

== matlab function data_collection_HILS/MATLAB Function8 ==
  settings: updateMethod=DISCRETE
  data: xyz_error input; window_size_ parameter; avg_array_xyz_error output
function avg_array_xyz_error  = fcn(xyz_error, window_size_)

coder.extrinsic('calculate_xyzerror.m');

% persistent 변수 선언
persistent initialized avg_array_xyz_error_;

% 초기화가 필요할 때만 실행
if isempty(initialized)
    initialized = true; % 초기화 완료 표시
    one_or_zero = 0;
    one_or_zero_ = 0;
    avg_array_xyz_error = 0.0;
    avg_array_xyz_error_ = 0.0;

    disp('initialized.');
end


[one_or_zero_, avg_array_xyz_error_] = calculate_xyzerror(xyz_error,window_size_);

one_or_zero = one_or_zero_;
avg_array_xyz_error = avg_array_xyz_error_;





end

== matlab function data_collection_HILS/MATLAB Function15 ==
  data: u input; y output
function y = fcn(u)
% HILS 환경에서는 전체 시뮬레이션 시간 동안 u의 최댓값을 찾습니다.

    coder.extrinsic('assignin');
    persistent max_val; % 최댓값을 저장할 변수

    % persistent 변수 초기화
    if isempty(max_val)
        max_val = -inf; % 처음에 매우 작은 값으로 초기화
    end

    % 현재 u가 기록된 최댓값보다 크면 업데이트
    if u > max_val
        max_val = u;
    end

    y = max_val; % 현재까지의 최댓값을 출력
    
    % 계산된 최댓값을 MATLAB Workspace 변수에 실시간으로 전송
    assignin('base', 'max_avg_xyz_error', y);

end

== matlab function data_collection_HILS/MATLAB Function1 ==
  data: pwm_in input; rad_s_out output
function rad_s_out = pwm_to_rads(pwm_in)
%#codegen

% 이 함수는 8x1 배열의 PWM 값을 입력받아
% 각 값을 rad/s 단위의 각속도로 변환합니다.

% --- 사용자 정의 파라미터 ---
% Gazebo SDF 파일 또는 PX4 파라미터에 맞춰 수정하세요.
maxRotVelocity = 425.47;  % rad/s
PWM_MIN = 1100;           % 시동(Armed) 시 최소 PWM 값
PWM_MAX = 2200;           % 최대 PWM 값
% -------------------------

% 출력 변수를 8x1 크기의 double 타입 배열로 초기화합니다.
rad_s_out = zeros(8, 1);

% 8개의 채널에 대해 반복 계산합니다.
for i = 1:8
    % 현재 채널의 PWM 값을 가져옵니다.
    % Simulink 입력은 종종 double 타입이므로, 먼저 double로 변환해줍니다.
    pwm_value = double(pwm_in(i));
    
    % 1. PWM 값을 0.0 ~ 1.0 사이의 정규화된 입력으로 변환
    % (pwm_value - PWM_MIN)이 음수가 되지 않도록 saturate 처리
    if pwm_value < PWM_MIN
        normalized_input = 0.0;
    elseif pwm_value > PWM_MAX
        normalized_input = 1.0;
    else
        normalized_input = (pwm_value - PWM_MIN) / (PWM_MAX - PWM_MIN);
    end
    
    % 2. 정규화된 입력을 rad/s로 변환
    rad_s_out(i) = normalized_input * maxRotVelocity;
end

end

== matlab function data_collection_HILS/MATLAB Function ==
  data: u input; y output
function y = fcn(u)
% HILS 환경에서는 전체 시뮬레이션 시간 동안 u의 최댓값을 찾습니다.

    coder.extrinsic('assignin');
    persistent max_val; % 최댓값을 저장할 변수

    % persistent 변수 초기화
    if isempty(max_val)
        max_val = -inf; % 처음에 매우 작은 값으로 초기화
    end

    % 현재 u가 기록된 최댓값보다 크면 업데이트
    if u > max_val
        max_val = u;
    end

    y = max_val; % 현재까지의 최댓값을 출력
    
    % 계산된 최댓값을 MATLAB Workspace 변수에 실시간으로 전송
    assignin('base', 'max_xy_error', y);

end

== matlab function data_collection_HILS/MATLAB Function2 ==
  data: endstep_z_error input; y output
function y = fcn(endstep_z_error)

% z_error 값을 기본 워크스페이스에 저장
assignin('base', 'endstep_z_error', endstep_z_error);

% 저장된 값을 반환
y = endstep_z_error;

end

== matlab function data_collection_HILS/MATLAB Function3 ==
  data: endstep_y_error input; y output
function y = fcn(endstep_y_error)

% z_error 값을 기본 워크스페이스에 저장
assignin('base', 'endstep_y_error', endstep_y_error);

% 저장된 값을 반환
y = endstep_y_error;

end

== matlab function data_collection_HILS/MATLAB Function4 ==
  data: endstep_x_error input; y output
function y = fcn(endstep_x_error)

% z_error 값을 기본 워크스페이스에 저장
assignin('base', 'endstep_x_error', endstep_x_error);

% 저장된 값을 반환
y = endstep_x_error;

end

== matlab function data_collection_HILS/MATLAB Function5 ==
  data: xy_error input; y output
function y = two_norm(xy_error)
    coder.extrinsic('norm'); % MATLAB 함수 사용을 알림
    
    

    
    % 'y'를 명확히 초기화
    y = 0; 
    
y = norm(xy_error,2);

== matlab function data_collection_HILS/MATLAB Function6 ==
  data: u input; y output
function y = fcn(u)
% HILS 환경에서는 전체 시뮬레이션 시간 동안 u의 최댓값을 찾습니다.

    coder.extrinsic('assignin');
    persistent max_val; % 최댓값을 저장할 변수

    % persistent 변수 초기화
    if isempty(max_val)
        max_val = -inf; % 처음에 매우 작은 값으로 초기화
    end

    % 현재 u가 기록된 최댓값보다 크면 업데이트
    if u > max_val
        max_val = u;
    end

    y = max_val; % 현재까지의 최댓값을 출력
    
    % 계산된 최댓값을 MATLAB Workspace 변수에 실시간으로 전송
    assignin('base', 'max_xy_error', y);

end

== matlab function data_collection_HILS/MATLAB Function7 ==
  data: u input; y output
function y = fcn(u)
% HILS 환경에서는 전체 시뮬레이션 시간 동안 u의 최댓값을 찾습니다.

    coder.extrinsic('assignin');
    persistent max_val; % 최댓값을 저장할 변수

    % persistent 변수 초기화
    if isempty(max_val)
        max_val = -inf; % 처음에 매우 작은 값으로 초기화
    end

    % 현재 u가 기록된 최댓값보다 크면 업데이트
    if u > max_val
        max_val = u;
    end

    y = max_val; % 현재까지의 최댓값을 출력
    
    % 계산된 최댓값을 MATLAB Workspace 변수에 실시간으로 전송
    assignin('base', 'max_xyz_error', y);

end

== matlab function data_collection_HILS/Subsystem2/MATLAB Function4 ==
  data: u input; y output
function y = fcn(u)
% HILS 환경에서는 전체 시뮬레이션 시간 동안 u의 절대값 최솟값을 찾습니다.

    coder.extrinsic('assignin');
    persistent min_val; % 최솟값을 저장할 변수

    % persistent 변수 초기화
    if isempty(min_val)
        min_val = inf; % 처음에 매우 큰 값으로 초기화
    end

    % 현재 u의 절대값이 기록된 최솟값보다 작으면 업데이트
    if abs(u) < min_val
        min_val = abs(u);
    end

    y = min_val; % 현재까지의 최솟값을 출력
    
    % 계산된 최솟값을 MATLAB Workspace 변수에 실시간으로 전송
    assignin('base', 'min_avg_array_FCM', y);

end

== matlab function data_collection_HILS/MATLAB Function9 ==
  data: endstep_xy_error input; y output
function y = fcn(endstep_xy_error)

% z_error 값을 기본 워크스페이스에 저장
assignin('base', 'endstep_xy_error', endstep_xy_error);

% 저장된 값을 반환
y = endstep_xy_error;

end
